simulink model "Practica_8_simulink"  (R2024b)
settings: Solver=VariableStepAuto  StartTime=0.0  StopTime=8  RelTol=1e-3
InitFcn:
  |     Ra=2;
  |     Kt=0.01;
  |     Ke=0.01;
  |     b=0.0012;
  |     La=0.023;
  |     J=0.001;
  |     T=0;
settings Model: Creator=newju

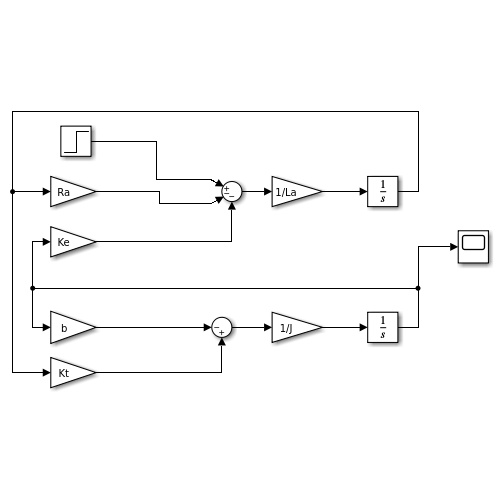
[thumbnail: Simulink's stored preview of the top-level diagram]
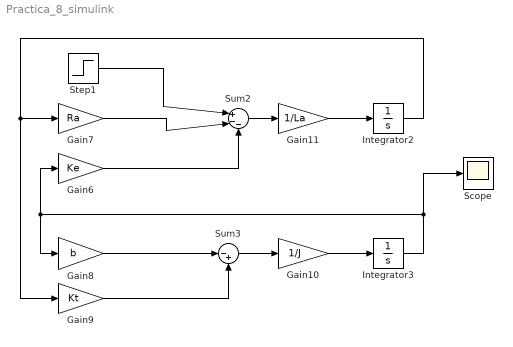
== system Practica_8_simulink ==
  Gain10 : Gain  Gain=1/J
  Gain11 : Gain  Gain=1/La
  Gain6 : Gain  Gain=Ke
  Gain7 : Gain  Gain=Ra
  Gain8 : Gain  Gain=b
  Gain9 : Gain  Gain=Kt
  Integrator2 : Integrator
  Integrator3 : Integrator
  Scope : Scope
  Step1 : Step  Time=0  After=5  SampleTime=0
  Sum2 : Sum  Inputs=|+--
  Sum3 : Sum  Inputs=|-+
  wires:
  Step1/1 -> Sum2/1
  Gain7/1 -> Sum2/2
  Gain6/1 -> Sum2/3
  Gain8/1 -> Sum3/1
  Gain9/1 -> Sum3/2
  Sum3/1 -> Gain10/1
  Sum2/1 -> Gain11/1
  Gain10/1 -> Integrator3/1
  Gain11/1 -> Integrator2/1
  Integrator3/1 -> Scope/1, Gain6/1, Gain8/1
  Integrator2/1 -> Gain7/1, Gain9/1
